simulink model "receiver_overall_reset"  (Simulink 7.5)
settings: Solver=FixedStepDiscrete  SolverMode=SingleTasking  StartTime=0.0  StopTime=(length(simin.signals.values)-1)/Fs  FixedStep=1  RelTol=1e-3
undefined symbols (not defined in the file): Fs
libraries: xbsIndex_r4 x962
(part 6 of 9)

== system receiver_overall_reset/Receiver/Sym-Clk/Corr/Delay_Line/DE16 ==
  In1 : Inport
  1to2 : Subsystem
  DE : xbsIndex_r4/Delay  en=off  latency=1  dbl_ovrd=off  reg_retiming=off  block_type=delay
      settings: xl_area=[1 1 0 0 0 0 0]  block_version=12.1
  Out1 : Outport
  Out2 : Outport  Port=2
  wires:
  1to2/2(Out2) -> Out2/1
  1to2/1(Out1) -> Out1/1
  In1/1 -> DE/1
  DE/1 -> 1to2/1(In)

== system receiver_overall_reset/Receiver/Sym-Clk/Corr/Delay_Line/DE17 ==
  In1 : Inport
  1to2 : Subsystem
  DE : xbsIndex_r4/Delay  en=off  latency=1  dbl_ovrd=off  reg_retiming=off  block_type=delay
      settings: xl_area=[1 1 0 0 0 0 0]  block_version=12.1
  Out1 : Outport
  Out2 : Outport  Port=2
  wires:
  1to2/2(Out2) -> Out2/1
  1to2/1(Out1) -> Out1/1
  In1/1 -> DE/1
  DE/1 -> 1to2/1(In)

== system receiver_overall_reset/Receiver/Sym-Clk/Corr/Delay_Line/DE18 ==
  In1 : Inport
  1to2 : Subsystem
  DE : xbsIndex_r4/Delay  en=off  latency=1  dbl_ovrd=off  reg_retiming=off  block_type=delay
      settings: xl_area=[1 1 0 0 0 0 0]  block_version=12.1
  Out1 : Outport
  Out2 : Outport  Port=2
  wires:
  1to2/2(Out2) -> Out2/1
  1to2/1(Out1) -> Out1/1
  In1/1 -> DE/1
  DE/1 -> 1to2/1(In)

== system receiver_overall_reset/Receiver/Sym-Clk/Corr/Delay_Line/DE19 ==
  In1 : Inport
  1to2 : Subsystem
  DE : xbsIndex_r4/Delay  en=off  latency=1  dbl_ovrd=off  reg_retiming=off  block_type=delay
      settings: xl_area=[1 1 0 0 0 0 0]  block_version=12.1
  Out1 : Outport
  Out2 : Outport  Port=2
  wires:
  1to2/2(Out2) -> Out2/1
  1to2/1(Out1) -> Out1/1
  In1/1 -> DE/1
  DE/1 -> 1to2/1(In)

== system receiver_overall_reset/Receiver/Sym-Clk/Corr/Delay_Line/DE2 ==
  In1 : Inport
  1to2 : Subsystem
  DE : xbsIndex_r4/Delay  en=off  latency=1  dbl_ovrd=off  reg_retiming=off  block_type=delay
      settings: xl_area=[1 1 0 0 0 0 0]  block_version=12.1
  Out1 : Outport
  Out2 : Outport  Port=2
  wires:
  1to2/2(Out2) -> Out2/1
  1to2/1(Out1) -> Out1/1
  In1/1 -> DE/1
  DE/1 -> 1to2/1(In)

== system receiver_overall_reset/Receiver/Sym-Clk/Corr/Delay_Line/DE20 ==
  In1 : Inport
  1to2 : Subsystem
  DE : xbsIndex_r4/Delay  en=off  latency=1  dbl_ovrd=off  reg_retiming=off  block_type=delay
      settings: xl_area=[1 1 0 0 0 0 0]  block_version=12.1
  Out1 : Outport
  Out2 : Outport  Port=2
  wires:
  1to2/2(Out2) -> Out2/1
  1to2/1(Out1) -> Out1/1
  In1/1 -> DE/1
  DE/1 -> 1to2/1(In)

== system receiver_overall_reset/Receiver/Sym-Clk/Corr/Delay_Line/DE21 ==
  In1 : Inport
  1to2 : Subsystem
  DE : xbsIndex_r4/Delay  en=off  latency=1  dbl_ovrd=off  reg_retiming=off  block_type=delay
      settings: xl_area=[1 1 0 0 0 0 0]  block_version=12.1
  Out1 : Outport
  Out2 : Outport  Port=2
  wires:
  1to2/2(Out2) -> Out2/1
  1to2/1(Out1) -> Out1/1
  In1/1 -> DE/1
  DE/1 -> 1to2/1(In)

== system receiver_overall_reset/Receiver/Sym-Clk/Corr/Delay_Line/DE22 ==
  In1 : Inport
  1to2 : Subsystem
  DE : xbsIndex_r4/Delay  en=off  latency=1  dbl_ovrd=off  reg_retiming=off  block_type=delay
      settings: xl_area=[1 1 0 0 0 0 0]  block_version=12.1
  Out1 : Outport
  Out2 : Outport  Port=2
  wires:
  1to2/2(Out2) -> Out2/1
  1to2/1(Out1) -> Out1/1
  In1/1 -> DE/1
  DE/1 -> 1to2/1(In)

== system receiver_overall_reset/Receiver/Sym-Clk/Corr/Delay_Line/DE23 ==
  In1 : Inport
  1to2 : Subsystem
  DE : xbsIndex_r4/Delay  en=off  latency=1  dbl_ovrd=off  reg_retiming=off  block_type=delay
      settings: xl_area=[1 1 0 0 0 0 0]  block_version=12.1
  Out1 : Outport
  Out2 : Outport  Port=2
  wires:
  1to2/2(Out2) -> Out2/1
  1to2/1(Out1) -> Out1/1
  In1/1 -> DE/1
  DE/1 -> 1to2/1(In)

== system receiver_overall_reset/Receiver/Sym-Clk/Corr/Delay_Line/DE24 ==
  In1 : Inport
  1to2 : Subsystem
  DE : xbsIndex_r4/Delay  en=off  latency=1  dbl_ovrd=off  reg_retiming=off  block_type=delay
      settings: xl_area=[1 1 0 0 0 0 0]  block_version=12.1
  Out1 : Outport
  Out2 : Outport  Port=2
  wires:
  1to2/2(Out2) -> Out2/1
  1to2/1(Out1) -> Out1/1
  In1/1 -> DE/1
  DE/1 -> 1to2/1(In)

== system receiver_overall_reset/Receiver/Sym-Clk/Corr/Delay_Line/DE25 ==
  In1 : Inport
  1to2 : Subsystem
  DE : xbsIndex_r4/Delay  en=off  latency=1  dbl_ovrd=off  reg_retiming=off  block_type=delay
      settings: xl_area=[1 1 0 0 0 0 0]  block_version=12.1
  Out1 : Outport
  Out2 : Outport  Port=2
  wires:
  1to2/2(Out2) -> Out2/1
  1to2/1(Out1) -> Out1/1
  In1/1 -> DE/1
  DE/1 -> 1to2/1(In)

== system receiver_overall_reset/Receiver/Sym-Clk/Corr/Delay_Line/DE26 ==
  In1 : Inport
  1to2 : Subsystem
  DE : xbsIndex_r4/Delay  en=off  latency=1  dbl_ovrd=off  reg_retiming=off  block_type=delay
      settings: xl_area=[1 1 0 0 0 0 0]  block_version=12.1
  Out1 : Outport
  Out2 : Outport  Port=2
  wires:
  1to2/2(Out2) -> Out2/1
  1to2/1(Out1) -> Out1/1
  In1/1 -> DE/1
  DE/1 -> 1to2/1(In)

== system receiver_overall_reset/Receiver/Sym-Clk/Corr/Delay_Line/DE27 ==
  In1 : Inport
  1to2 : Subsystem
  DE : xbsIndex_r4/Delay  en=off  latency=1  dbl_ovrd=off  reg_retiming=off  block_type=delay
      settings: xl_area=[1 1 0 0 0 0 0]  block_version=12.1
  Out1 : Outport
  Out2 : Outport  Port=2
  wires:
  1to2/2(Out2) -> Out2/1
  1to2/1(Out1) -> Out1/1
  In1/1 -> DE/1
  DE/1 -> 1to2/1(In)

== system receiver_overall_reset/Receiver/Sym-Clk/Corr/Delay_Line/DE28 ==
  In1 : Inport
  1to2 : Subsystem
  DE : xbsIndex_r4/Delay  en=off  latency=1  dbl_ovrd=off  reg_retiming=off  block_type=delay
      settings: xl_area=[1 1 0 0 0 0 0]  block_version=12.1
  Out1 : Outport
  Out2 : Outport  Port=2
  wires:
  1to2/2(Out2) -> Out2/1
  1to2/1(Out1) -> Out1/1
  In1/1 -> DE/1
  DE/1 -> 1to2/1(In)

== system receiver_overall_reset/Receiver/Sym-Clk/Corr/Delay_Line/DE29 ==
  In1 : Inport
  1to2 : Subsystem
  DE : xbsIndex_r4/Delay  en=off  latency=1  dbl_ovrd=off  reg_retiming=off  block_type=delay
      settings: xl_area=[1 1 0 0 0 0 0]  block_version=12.1
  Out1 : Outport
  Out2 : Outport  Port=2
  wires:
  1to2/2(Out2) -> Out2/1
  1to2/1(Out1) -> Out1/1
  In1/1 -> DE/1
  DE/1 -> 1to2/1(In)

== system receiver_overall_reset/Receiver/Sym-Clk/Corr/Delay_Line/DE3 ==
  In1 : Inport
  1to2 : Subsystem
  DE : xbsIndex_r4/Delay  en=off  latency=1  dbl_ovrd=off  reg_retiming=off  block_type=delay
      settings: xl_area=[1 1 0 0 0 0 0]  block_version=12.1
  Out1 : Outport
  Out2 : Outport  Port=2
  wires:
  1to2/2(Out2) -> Out2/1
  1to2/1(Out1) -> Out1/1
  In1/1 -> DE/1
  DE/1 -> 1to2/1(In)

== system receiver_overall_reset/Receiver/Sym-Clk/Corr/Delay_Line/DE30 ==
  In1 : Inport
  1to2 : Subsystem
  DE : xbsIndex_r4/Delay  en=off  latency=1  dbl_ovrd=off  reg_retiming=off  block_type=delay
      settings: xl_area=[1 1 0 0 0 0 0]  block_version=12.1
  Out1 : Outport
  Out2 : Outport  Port=2
  wires:
  1to2/2(Out2) -> Out2/1
  1to2/1(Out1) -> Out1/1
  In1/1 -> DE/1
  DE/1 -> 1to2/1(In)

== system receiver_overall_reset/Receiver/Sym-Clk/Corr/Delay_Line/DE4 ==
  In1 : Inport
  1to2 : Subsystem
  DE : xbsIndex_r4/Delay  en=off  latency=1  dbl_ovrd=off  reg_retiming=off  block_type=delay
      settings: xl_area=[1 1 0 0 0 0 0]  block_version=12.1
  Out1 : Outport
  Out2 : Outport  Port=2
  wires:
  1to2/2(Out2) -> Out2/1
  1to2/1(Out1) -> Out1/1
  In1/1 -> DE/1
  DE/1 -> 1to2/1(In)

== system receiver_overall_reset/Receiver/Sym-Clk/Corr/Delay_Line/DE5 ==
  In1 : Inport
  1to2 : Subsystem
  DE : xbsIndex_r4/Delay  en=off  latency=1  dbl_ovrd=off  reg_retiming=off  block_type=delay
      settings: xl_area=[1 1 0 0 0 0 0]  block_version=12.1
  Out1 : Outport
  Out2 : Outport  Port=2
  wires:
  1to2/2(Out2) -> Out2/1
  1to2/1(Out1) -> Out1/1
  In1/1 -> DE/1
  DE/1 -> 1to2/1(In)

== system receiver_overall_reset/Receiver/Sym-Clk/Corr/Delay_Line/DE6 ==
  In1 : Inport
  1to2 : Subsystem
  DE : xbsIndex_r4/Delay  en=off  latency=1  dbl_ovrd=off  reg_retiming=off  block_type=delay
      settings: xl_area=[1 1 0 0 0 0 0]  block_version=12.1
  Out1 : Outport
  Out2 : Outport  Port=2
  wires:
  1to2/2(Out2) -> Out2/1
  1to2/1(Out1) -> Out1/1
  In1/1 -> DE/1
  DE/1 -> 1to2/1(In)

== system receiver_overall_reset/Receiver/Sym-Clk/Corr/Delay_Line/DE7 ==
  In1 : Inport
  1to2 : Subsystem
  DE : xbsIndex_r4/Delay  en=off  latency=1  dbl_ovrd=off  reg_retiming=off  block_type=delay
      settings: xl_area=[1 1 0 0 0 0 0]  block_version=12.1
  Out1 : Outport
  Out2 : Outport  Port=2
  wires:
  1to2/2(Out2) -> Out2/1
  1to2/1(Out1) -> Out1/1
  In1/1 -> DE/1
  DE/1 -> 1to2/1(In)

== system receiver_overall_reset/Receiver/Sym-Clk/Corr/Delay_Line/DE8 ==
  In1 : Inport
  1to2 : Subsystem
  DE : xbsIndex_r4/Delay  en=off  latency=1  dbl_ovrd=off  reg_retiming=off  block_type=delay
      settings: xl_area=[1 1 0 0 0 0 0]  block_version=12.1
  Out1 : Outport
  Out2 : Outport  Port=2
  wires:
  1to2/2(Out2) -> Out2/1
  1to2/1(Out1) -> Out1/1
  In1/1 -> DE/1
  DE/1 -> 1to2/1(In)

== system receiver_overall_reset/Receiver/Sym-Clk/Corr/Delay_Line/DE9 ==
  In1 : Inport
  1to2 : Subsystem
  DE : xbsIndex_r4/Delay  en=off  latency=1  dbl_ovrd=off  reg_retiming=off  block_type=delay
      settings: xl_area=[1 1 0 0 0 0 0]  block_version=12.1
  Out1 : Outport
  Out2 : Outport  Port=2
  wires:
  1to2/2(Out2) -> Out2/1
  1to2/1(Out1) -> Out1/1
  In1/1 -> DE/1
  DE/1 -> 1to2/1(In)

== system receiver_overall_reset/Receiver/Sym-Chooser/0-8/Corr0/Delay_Line/1to2 ==
  In : Inport  OutDataType=fixdt(1, 16)  OutScaling=2^0
  Out1 : Outport  OutDataType=fixdt(1, 16)  OutScaling=2^0
  Out2 : Outport  Port=2  OutDataType=fixdt(1, 16)  OutScaling=2^0
  wires:
  In/1 -> Out1/1, Out2/1

== system receiver_overall_reset/Receiver/Sym-Chooser/0-8/Corr0/Delay_Line/DE1 ==
  In1 : Inport
  1to2 : Subsystem
  DE : xbsIndex_r4/Delay  en=off  latency=1  dbl_ovrd=off  reg_retiming=off  block_type=delay
      settings: xl_area=[1 1 0 0 0 0 0]  block_version=12.1
  Out1 : Outport
  Out2 : Outport  Port=2
  wires:
  DE/1 -> 1to2/1(In)
  In1/1 -> DE/1
  1to2/1(Out1) -> Out1/1
  1to2/2(Out2) -> Out2/1

== system receiver_overall_reset/Receiver/Sym-Chooser/0-8/Corr0/Delay_Line/DE10 ==
  In1 : Inport
  1to2 : Subsystem
  DE : xbsIndex_r4/Delay  en=off  latency=1  dbl_ovrd=off  reg_retiming=off  block_type=delay
      settings: xl_area=[1 1 0 0 0 0 0]  block_version=12.1
  Out1 : Outport
  Out2 : Outport  Port=2
  wires:
  1to2/2(Out2) -> Out2/1
  1to2/1(Out1) -> Out1/1
  In1/1 -> DE/1
  DE/1 -> 1to2/1(In)

== system receiver_overall_reset/Receiver/Sym-Chooser/0-8/Corr0/Delay_Line/DE11 ==
  In1 : Inport
  1to2 : Subsystem
  DE : xbsIndex_r4/Delay  en=off  latency=1  dbl_ovrd=off  reg_retiming=off  block_type=delay
      settings: xl_area=[1 1 0 0 0 0 0]  block_version=12.1
  Out1 : Outport
  Out2 : Outport  Port=2
  wires:
  1to2/2(Out2) -> Out2/1
  1to2/1(Out1) -> Out1/1
  In1/1 -> DE/1
  DE/1 -> 1to2/1(In)

== system receiver_overall_reset/Receiver/Sym-Chooser/0-8/Corr0/Delay_Line/DE12 ==
  In1 : Inport
  1to2 : Subsystem
  DE : xbsIndex_r4/Delay  en=off  latency=1  dbl_ovrd=off  reg_retiming=off  block_type=delay
      settings: xl_area=[1 1 0 0 0 0 0]  block_version=12.1
  Out1 : Outport
  Out2 : Outport  Port=2
  wires:
  1to2/2(Out2) -> Out2/1
  1to2/1(Out1) -> Out1/1
  In1/1 -> DE/1
  DE/1 -> 1to2/1(In)

== system receiver_overall_reset/Receiver/Sym-Chooser/0-8/Corr0/Delay_Line/DE13 ==
  In1 : Inport
  1to2 : Subsystem
  DE : xbsIndex_r4/Delay  en=off  latency=1  dbl_ovrd=off  reg_retiming=off  block_type=delay
      settings: xl_area=[1 1 0 0 0 0 0]  block_version=12.1
  Out1 : Outport
  Out2 : Outport  Port=2
  wires:
  1to2/2(Out2) -> Out2/1
  1to2/1(Out1) -> Out1/1
  In1/1 -> DE/1
  DE/1 -> 1to2/1(In)

== system receiver_overall_reset/Receiver/Sym-Chooser/0-8/Corr0/Delay_Line/DE14 ==
  In1 : Inport
  1to2 : Subsystem
  DE : xbsIndex_r4/Delay  en=off  latency=1  dbl_ovrd=off  reg_retiming=off  block_type=delay
      settings: xl_area=[1 1 0 0 0 0 0]  block_version=12.1
  Out1 : Outport
  Out2 : Outport  Port=2
  wires:
  1to2/2(Out2) -> Out2/1
  1to2/1(Out1) -> Out1/1
  In1/1 -> DE/1
  DE/1 -> 1to2/1(In)

== system receiver_overall_reset/Receiver/Sym-Chooser/0-8/Corr0/Delay_Line/DE15 ==
  In1 : Inport
  1to2 : Subsystem
  DE : xbsIndex_r4/Delay  en=off  latency=1  dbl_ovrd=off  reg_retiming=off  block_type=delay
      settings: xl_area=[1 1 0 0 0 0 0]  block_version=12.1
  Out1 : Outport
  Out2 : Outport  Port=2
  wires:
  1to2/2(Out2) -> Out2/1
  1to2/1(Out1) -> Out1/1
  In1/1 -> DE/1
  DE/1 -> 1to2/1(In)

== system receiver_overall_reset/Receiver/Sym-Chooser/0-8/Corr0/Delay_Line/DE16 ==
  In1 : Inport
  1to2 : Subsystem
  DE : xbsIndex_r4/Delay  en=off  latency=1  dbl_ovrd=off  reg_retiming=off  block_type=delay
      settings: xl_area=[1 1 0 0 0 0 0]  block_version=12.1
  Out1 : Outport
  Out2 : Outport  Port=2
  wires:
  1to2/2(Out2) -> Out2/1
  1to2/1(Out1) -> Out1/1
  In1/1 -> DE/1
  DE/1 -> 1to2/1(In)

== system receiver_overall_reset/Receiver/Sym-Chooser/0-8/Corr0/Delay_Line/DE17 ==
  In1 : Inport
  1to2 : Subsystem
  DE : xbsIndex_r4/Delay  en=off  latency=1  dbl_ovrd=off  reg_retiming=off  block_type=delay
      settings: xl_area=[1 1 0 0 0 0 0]  block_version=12.1
  Out1 : Outport
  Out2 : Outport  Port=2
  wires:
  1to2/2(Out2) -> Out2/1
  1to2/1(Out1) -> Out1/1
  In1/1 -> DE/1
  DE/1 -> 1to2/1(In)

== system receiver_overall_reset/Receiver/Sym-Chooser/0-8/Corr0/Delay_Line/DE18 ==
  In1 : Inport
  1to2 : Subsystem
  DE : xbsIndex_r4/Delay  en=off  latency=1  dbl_ovrd=off  reg_retiming=off  block_type=delay
      settings: xl_area=[1 1 0 0 0 0 0]  block_version=12.1
  Out1 : Outport
  Out2 : Outport  Port=2
  wires:
  1to2/2(Out2) -> Out2/1
  1to2/1(Out1) -> Out1/1
  In1/1 -> DE/1
  DE/1 -> 1to2/1(In)

== system receiver_overall_reset/Receiver/Sym-Chooser/0-8/Corr0/Delay_Line/DE19 ==
  In1 : Inport
  1to2 : Subsystem
  DE : xbsIndex_r4/Delay  en=off  latency=1  dbl_ovrd=off  reg_retiming=off  block_type=delay
      settings: xl_area=[1 1 0 0 0 0 0]  block_version=12.1
  Out1 : Outport
  Out2 : Outport  Port=2
  wires:
  1to2/2(Out2) -> Out2/1
  1to2/1(Out1) -> Out1/1
  In1/1 -> DE/1
  DE/1 -> 1to2/1(In)

== system receiver_overall_reset/Receiver/Sym-Chooser/0-8/Corr0/Delay_Line/DE2 ==
  In1 : Inport
  1to2 : Subsystem
  DE : xbsIndex_r4/Delay  en=off  latency=1  dbl_ovrd=off  reg_retiming=off  block_type=delay
      settings: xl_area=[1 1 0 0 0 0 0]  block_version=12.1
  Out1 : Outport
  Out2 : Outport  Port=2
  wires:
  1to2/2(Out2) -> Out2/1
  1to2/1(Out1) -> Out1/1
  In1/1 -> DE/1
  DE/1 -> 1to2/1(In)

== system receiver_overall_reset/Receiver/Sym-Chooser/0-8/Corr0/Delay_Line/DE20 ==
  In1 : Inport
  1to2 : Subsystem
  DE : xbsIndex_r4/Delay  en=off  latency=1  dbl_ovrd=off  reg_retiming=off  block_type=delay
      settings: xl_area=[1 1 0 0 0 0 0]  block_version=12.1
  Out1 : Outport
  Out2 : Outport  Port=2
  wires:
  1to2/2(Out2) -> Out2/1
  1to2/1(Out1) -> Out1/1
  In1/1 -> DE/1
  DE/1 -> 1to2/1(In)

== system receiver_overall_reset/Receiver/Sym-Chooser/0-8/Corr0/Delay_Line/DE21 ==
  In1 : Inport
  1to2 : Subsystem
  DE : xbsIndex_r4/Delay  en=off  latency=1  dbl_ovrd=off  reg_retiming=off  block_type=delay
      settings: xl_area=[1 1 0 0 0 0 0]  block_version=12.1
  Out1 : Outport
  Out2 : Outport  Port=2
  wires:
  1to2/2(Out2) -> Out2/1
  1to2/1(Out1) -> Out1/1
  In1/1 -> DE/1
  DE/1 -> 1to2/1(In)

== system receiver_overall_reset/Receiver/Sym-Chooser/0-8/Corr0/Delay_Line/DE22 ==
  In1 : Inport
  1to2 : Subsystem
  DE : xbsIndex_r4/Delay  en=off  latency=1  dbl_ovrd=off  reg_retiming=off  block_type=delay
      settings: xl_area=[1 1 0 0 0 0 0]  block_version=12.1
  Out1 : Outport
  Out2 : Outport  Port=2
  wires:
  1to2/2(Out2) -> Out2/1
  1to2/1(Out1) -> Out1/1
  In1/1 -> DE/1
  DE/1 -> 1to2/1(In)

== system receiver_overall_reset/Receiver/Sym-Chooser/0-8/Corr0/Delay_Line/DE23 ==
  In1 : Inport
  1to2 : Subsystem
  DE : xbsIndex_r4/Delay  en=off  latency=1  dbl_ovrd=off  reg_retiming=off  block_type=delay
      settings: xl_area=[1 1 0 0 0 0 0]  block_version=12.1
  Out1 : Outport
  Out2 : Outport  Port=2
  wires:
  1to2/2(Out2) -> Out2/1
  1to2/1(Out1) -> Out1/1
  In1/1 -> DE/1
  DE/1 -> 1to2/1(In)

== system receiver_overall_reset/Receiver/Sym-Chooser/0-8/Corr0/Delay_Line/DE24 ==
  In1 : Inport
  1to2 : Subsystem
  DE : xbsIndex_r4/Delay  en=off  latency=1  dbl_ovrd=off  reg_retiming=off  block_type=delay
      settings: xl_area=[1 1 0 0 0 0 0]  block_version=12.1
  Out1 : Outport
  Out2 : Outport  Port=2
  wires:
  1to2/2(Out2) -> Out2/1
  1to2/1(Out1) -> Out1/1
  In1/1 -> DE/1
  DE/1 -> 1to2/1(In)

== system receiver_overall_reset/Receiver/Sym-Chooser/0-8/Corr0/Delay_Line/DE25 ==
  In1 : Inport
  1to2 : Subsystem
  DE : xbsIndex_r4/Delay  en=off  latency=1  dbl_ovrd=off  reg_retiming=off  block_type=delay
      settings: xl_area=[1 1 0 0 0 0 0]  block_version=12.1
  Out1 : Outport
  Out2 : Outport  Port=2
  wires:
  1to2/2(Out2) -> Out2/1
  1to2/1(Out1) -> Out1/1
  In1/1 -> DE/1
  DE/1 -> 1to2/1(In)

== system receiver_overall_reset/Receiver/Sym-Chooser/0-8/Corr0/Delay_Line/DE26 ==
  In1 : Inport
  1to2 : Subsystem
  DE : xbsIndex_r4/Delay  en=off  latency=1  dbl_ovrd=off  reg_retiming=off  block_type=delay
      settings: xl_area=[1 1 0 0 0 0 0]  block_version=12.1
  Out1 : Outport
  Out2 : Outport  Port=2
  wires:
  1to2/2(Out2) -> Out2/1
  1to2/1(Out1) -> Out1/1
  In1/1 -> DE/1
  DE/1 -> 1to2/1(In)

== system receiver_overall_reset/Receiver/Sym-Chooser/0-8/Corr0/Delay_Line/DE27 ==
  In1 : Inport
  1to2 : Subsystem
  DE : xbsIndex_r4/Delay  en=off  latency=1  dbl_ovrd=off  reg_retiming=off  block_type=delay
      settings: xl_area=[1 1 0 0 0 0 0]  block_version=12.1
  Out1 : Outport
  Out2 : Outport  Port=2
  wires:
  1to2/2(Out2) -> Out2/1
  1to2/1(Out1) -> Out1/1
  In1/1 -> DE/1
  DE/1 -> 1to2/1(In)

== system receiver_overall_reset/Receiver/Sym-Chooser/0-8/Corr0/Delay_Line/DE28 ==
  In1 : Inport
  1to2 : Subsystem
  DE : xbsIndex_r4/Delay  en=off  latency=1  dbl_ovrd=off  reg_retiming=off  block_type=delay
      settings: xl_area=[1 1 0 0 0 0 0]  block_version=12.1
  Out1 : Outport
  Out2 : Outport  Port=2
  wires:
  1to2/2(Out2) -> Out2/1
  1to2/1(Out1) -> Out1/1
  In1/1 -> DE/1
  DE/1 -> 1to2/1(In)

== system receiver_overall_reset/Receiver/Sym-Chooser/0-8/Corr0/Delay_Line/DE29 ==
  In1 : Inport
  1to2 : Subsystem
  DE : xbsIndex_r4/Delay  en=off  latency=1  dbl_ovrd=off  reg_retiming=off  block_type=delay
      settings: xl_area=[1 1 0 0 0 0 0]  block_version=12.1
  Out1 : Outport
  Out2 : Outport  Port=2
  wires:
  1to2/2(Out2) -> Out2/1
  1to2/1(Out1) -> Out1/1
  In1/1 -> DE/1
  DE/1 -> 1to2/1(In)

== system receiver_overall_reset/Receiver/Sym-Chooser/0-8/Corr0/Delay_Line/DE3 ==
  In1 : Inport
  1to2 : Subsystem
  DE : xbsIndex_r4/Delay  en=off  latency=1  dbl_ovrd=off  reg_retiming=off  block_type=delay
      settings: xl_area=[1 1 0 0 0 0 0]  block_version=12.1
  Out1 : Outport
  Out2 : Outport  Port=2
  wires:
  1to2/2(Out2) -> Out2/1
  1to2/1(Out1) -> Out1/1
  In1/1 -> DE/1
  DE/1 -> 1to2/1(In)

== system receiver_overall_reset/Receiver/Sym-Chooser/0-8/Corr0/Delay_Line/DE30 ==
  In1 : Inport
  1to2 : Subsystem
  DE : xbsIndex_r4/Delay  en=off  latency=1  dbl_ovrd=off  reg_retiming=off  block_type=delay
      settings: xl_area=[1 1 0 0 0 0 0]  block_version=12.1
  Out1 : Outport
  Out2 : Outport  Port=2
  wires:
  1to2/2(Out2) -> Out2/1
  1to2/1(Out1) -> Out1/1
  In1/1 -> DE/1
  DE/1 -> 1to2/1(In)

== system receiver_overall_reset/Receiver/Sym-Chooser/0-8/Corr0/Delay_Line/DE4 ==
  In1 : Inport
  1to2 : Subsystem
  DE : xbsIndex_r4/Delay  en=off  latency=1  dbl_ovrd=off  reg_retiming=off  block_type=delay
      settings: xl_area=[1 1 0 0 0 0 0]  block_version=12.1
  Out1 : Outport
  Out2 : Outport  Port=2
  wires:
  1to2/2(Out2) -> Out2/1
  1to2/1(Out1) -> Out1/1
  In1/1 -> DE/1
  DE/1 -> 1to2/1(In)

== system receiver_overall_reset/Receiver/Sym-Chooser/0-8/Corr0/Delay_Line/DE5 ==
  In1 : Inport
  1to2 : Subsystem
  DE : xbsIndex_r4/Delay  en=off  latency=1  dbl_ovrd=off  reg_retiming=off  block_type=delay
      settings: xl_area=[1 1 0 0 0 0 0]  block_version=12.1
  Out1 : Outport
  Out2 : Outport  Port=2
  wires:
  1to2/2(Out2) -> Out2/1
  1to2/1(Out1) -> Out1/1
  In1/1 -> DE/1
  DE/1 -> 1to2/1(In)

== system receiver_overall_reset/Receiver/Sym-Chooser/0-8/Corr0/Delay_Line/DE6 ==
  In1 : Inport
  1to2 : Subsystem
  DE : xbsIndex_r4/Delay  en=off  latency=1  dbl_ovrd=off  reg_retiming=off  block_type=delay
      settings: xl_area=[1 1 0 0 0 0 0]  block_version=12.1
  Out1 : Outport
  Out2 : Outport  Port=2
  wires:
  1to2/2(Out2) -> Out2/1
  1to2/1(Out1) -> Out1/1
  In1/1 -> DE/1
  DE/1 -> 1to2/1(In)

== system receiver_overall_reset/Receiver/Sym-Chooser/0-8/Corr0/Delay_Line/DE7 ==
  In1 : Inport
  1to2 : Subsystem
  DE : xbsIndex_r4/Delay  en=off  latency=1  dbl_ovrd=off  reg_retiming=off  block_type=delay
      settings: xl_area=[1 1 0 0 0 0 0]  block_version=12.1
  Out1 : Outport
  Out2 : Outport  Port=2
  wires:
  1to2/2(Out2) -> Out2/1
  1to2/1(Out1) -> Out1/1
  In1/1 -> DE/1
  DE/1 -> 1to2/1(In)

== system receiver_overall_reset/Receiver/Sym-Chooser/0-8/Corr0/Delay_Line/DE8 ==
  In1 : Inport
  1to2 : Subsystem
  DE : xbsIndex_r4/Delay  en=off  latency=1  dbl_ovrd=off  reg_retiming=off  block_type=delay
      settings: xl_area=[1 1 0 0 0 0 0]  block_version=12.1
  Out1 : Outport
  Out2 : Outport  Port=2
  wires:
  1to2/2(Out2) -> Out2/1
  1to2/1(Out1) -> Out1/1
  In1/1 -> DE/1
  DE/1 -> 1to2/1(In)

== system receiver_overall_reset/Receiver/Sym-Chooser/0-8/Corr0/Delay_Line/DE9 ==
  In1 : Inport
  1to2 : Subsystem
  DE : xbsIndex_r4/Delay  en=off  latency=1  dbl_ovrd=off  reg_retiming=off  block_type=delay
      settings: xl_area=[1 1 0 0 0 0 0]  block_version=12.1
  Out1 : Outport
  Out2 : Outport  Port=2
  wires:
  1to2/2(Out2) -> Out2/1
  1to2/1(Out1) -> Out1/1
  In1/1 -> DE/1
  DE/1 -> 1to2/1(In)

== system receiver_overall_reset/Receiver/Sym-Chooser/1-9/Corr0/Delay_Line/1to2 ==
  In : Inport  OutDataType=fixdt(1, 16)  OutScaling=2^0
  Out1 : Outport  OutDataType=fixdt(1, 16)  OutScaling=2^0
  Out2 : Outport  Port=2  OutDataType=fixdt(1, 16)  OutScaling=2^0
  wires:
  In/1 -> Out1/1, Out2/1

== system receiver_overall_reset/Receiver/Sym-Chooser/1-9/Corr0/Delay_Line/DE1 ==
  In1 : Inport
  1to2 : Subsystem
  DE : xbsIndex_r4/Delay  en=off  latency=1  dbl_ovrd=off  reg_retiming=off  block_type=delay
      settings: xl_area=[1 1 0 0 0 0 0]  block_version=12.1
  Out1 : Outport
  Out2 : Outport  Port=2
  wires:
  DE/1 -> 1to2/1(In)
  In1/1 -> DE/1
  1to2/1(Out1) -> Out1/1
  1to2/2(Out2) -> Out2/1

== system receiver_overall_reset/Receiver/Sym-Chooser/1-9/Corr0/Delay_Line/DE10 ==
  In1 : Inport
  1to2 : Subsystem
  DE : xbsIndex_r4/Delay  en=off  latency=1  dbl_ovrd=off  reg_retiming=off  block_type=delay
      settings: xl_area=[1 1 0 0 0 0 0]  block_version=12.1
  Out1 : Outport
  Out2 : Outport  Port=2
  wires:
  1to2/2(Out2) -> Out2/1
  1to2/1(Out1) -> Out1/1
  In1/1 -> DE/1
  DE/1 -> 1to2/1(In)

== system receiver_overall_reset/Receiver/Sym-Chooser/1-9/Corr0/Delay_Line/DE11 ==
  In1 : Inport
  1to2 : Subsystem
  DE : xbsIndex_r4/Delay  en=off  latency=1  dbl_ovrd=off  reg_retiming=off  block_type=delay
      settings: xl_area=[1 1 0 0 0 0 0]  block_version=12.1
  Out1 : Outport
  Out2 : Outport  Port=2
  wires:
  1to2/2(Out2) -> Out2/1
  1to2/1(Out1) -> Out1/1
  In1/1 -> DE/1
  DE/1 -> 1to2/1(In)

== system receiver_overall_reset/Receiver/Sym-Chooser/1-9/Corr0/Delay_Line/DE12 ==
  In1 : Inport
  1to2 : Subsystem
  DE : xbsIndex_r4/Delay  en=off  latency=1  dbl_ovrd=off  reg_retiming=off  block_type=delay
      settings: xl_area=[1 1 0 0 0 0 0]  block_version=12.1
  Out1 : Outport
  Out2 : Outport  Port=2
  wires:
  1to2/2(Out2) -> Out2/1
  1to2/1(Out1) -> Out1/1
  In1/1 -> DE/1
  DE/1 -> 1to2/1(In)

== system receiver_overall_reset/Receiver/Sym-Chooser/1-9/Corr0/Delay_Line/DE13 ==
  In1 : Inport
  1to2 : Subsystem
  DE : xbsIndex_r4/Delay  en=off  latency=1  dbl_ovrd=off  reg_retiming=off  block_type=delay
      settings: xl_area=[1 1 0 0 0 0 0]  block_version=12.1
  Out1 : Outport
  Out2 : Outport  Port=2
  wires:
  1to2/2(Out2) -> Out2/1
  1to2/1(Out1) -> Out1/1
  In1/1 -> DE/1
  DE/1 -> 1to2/1(In)

== system receiver_overall_reset/Receiver/Sym-Chooser/1-9/Corr0/Delay_Line/DE14 ==
  In1 : Inport
  1to2 : Subsystem
  DE : xbsIndex_r4/Delay  en=off  latency=1  dbl_ovrd=off  reg_retiming=off  block_type=delay
      settings: xl_area=[1 1 0 0 0 0 0]  block_version=12.1
  Out1 : Outport
  Out2 : Outport  Port=2
  wires:
  1to2/2(Out2) -> Out2/1
  1to2/1(Out1) -> Out1/1
  In1/1 -> DE/1
  DE/1 -> 1to2/1(In)

== system receiver_overall_reset/Receiver/Sym-Chooser/1-9/Corr0/Delay_Line/DE15 ==
  In1 : Inport
  1to2 : Subsystem
  DE : xbsIndex_r4/Delay  en=off  latency=1  dbl_ovrd=off  reg_retiming=off  block_type=delay
      settings: xl_area=[1 1 0 0 0 0 0]  block_version=12.1
  Out1 : Outport
  Out2 : Outport  Port=2
  wires:
  1to2/2(Out2) -> Out2/1
  1to2/1(Out1) -> Out1/1
  In1/1 -> DE/1
  DE/1 -> 1to2/1(In)

== system receiver_overall_reset/Receiver/Sym-Chooser/1-9/Corr0/Delay_Line/DE16 ==
  In1 : Inport
  1to2 : Subsystem
  DE : xbsIndex_r4/Delay  en=off  latency=1  dbl_ovrd=off  reg_retiming=off  block_type=delay
      settings: xl_area=[1 1 0 0 0 0 0]  block_version=12.1
  Out1 : Outport
  Out2 : Outport  Port=2
  wires:
  1to2/2(Out2) -> Out2/1
  1to2/1(Out1) -> Out1/1
  In1/1 -> DE/1
  DE/1 -> 1to2/1(In)

== system receiver_overall_reset/Receiver/Sym-Chooser/1-9/Corr0/Delay_Line/DE17 ==
  In1 : Inport
  1to2 : Subsystem
  DE : xbsIndex_r4/Delay  en=off  latency=1  dbl_ovrd=off  reg_retiming=off  block_type=delay
      settings: xl_area=[1 1 0 0 0 0 0]  block_version=12.1
  Out1 : Outport
  Out2 : Outport  Port=2
  wires:
  1to2/2(Out2) -> Out2/1
  1to2/1(Out1) -> Out1/1
  In1/1 -> DE/1
  DE/1 -> 1to2/1(In)

== system receiver_overall_reset/Receiver/Sym-Chooser/1-9/Corr0/Delay_Line/DE18 ==
  In1 : Inport
  1to2 : Subsystem
  DE : xbsIndex_r4/Delay  en=off  latency=1  dbl_ovrd=off  reg_retiming=off  block_type=delay
      settings: xl_area=[1 1 0 0 0 0 0]  block_version=12.1
  Out1 : Outport
  Out2 : Outport  Port=2
  wires:
  1to2/2(Out2) -> Out2/1
  1to2/1(Out1) -> Out1/1
  In1/1 -> DE/1
  DE/1 -> 1to2/1(In)

== system receiver_overall_reset/Receiver/Sym-Chooser/1-9/Corr0/Delay_Line/DE19 ==
  In1 : Inport
  1to2 : Subsystem
  DE : xbsIndex_r4/Delay  en=off  latency=1  dbl_ovrd=off  reg_retiming=off  block_type=delay
      settings: xl_area=[1 1 0 0 0 0 0]  block_version=12.1
  Out1 : Outport
  Out2 : Outport  Port=2
  wires:
  1to2/2(Out2) -> Out2/1
  1to2/1(Out1) -> Out1/1
  In1/1 -> DE/1
  DE/1 -> 1to2/1(In)

== system receiver_overall_reset/Receiver/Sym-Chooser/1-9/Corr0/Delay_Line/DE2 ==
  In1 : Inport
  1to2 : Subsystem
  DE : xbsIndex_r4/Delay  en=off  latency=1  dbl_ovrd=off  reg_retiming=off  block_type=delay
      settings: xl_area=[1 1 0 0 0 0 0]  block_version=12.1
  Out1 : Outport
  Out2 : Outport  Port=2
  wires:
  1to2/2(Out2) -> Out2/1
  1to2/1(Out1) -> Out1/1
  In1/1 -> DE/1
  DE/1 -> 1to2/1(In)

== system receiver_overall_reset/Receiver/Sym-Chooser/1-9/Corr0/Delay_Line/DE20 ==
  In1 : Inport
  1to2 : Subsystem
  DE : xbsIndex_r4/Delay  en=off  latency=1  dbl_ovrd=off  reg_retiming=off  block_type=delay
      settings: xl_area=[1 1 0 0 0 0 0]  block_version=12.1
  Out1 : Outport
  Out2 : Outport  Port=2
  wires:
  1to2/2(Out2) -> Out2/1
  1to2/1(Out1) -> Out1/1
  In1/1 -> DE/1
  DE/1 -> 1to2/1(In)

== system receiver_overall_reset/Receiver/Sym-Chooser/1-9/Corr0/Delay_Line/DE21 ==
  In1 : Inport
  1to2 : Subsystem
  DE : xbsIndex_r4/Delay  en=off  latency=1  dbl_ovrd=off  reg_retiming=off  block_type=delay
      settings: xl_area=[1 1 0 0 0 0 0]  block_version=12.1
  Out1 : Outport
  Out2 : Outport  Port=2
  wires:
  1to2/2(Out2) -> Out2/1
  1to2/1(Out1) -> Out1/1
  In1/1 -> DE/1
  DE/1 -> 1to2/1(In)

== system receiver_overall_reset/Receiver/Sym-Chooser/1-9/Corr0/Delay_Line/DE22 ==
  In1 : Inport
  1to2 : Subsystem
  DE : xbsIndex_r4/Delay  en=off  latency=1  dbl_ovrd=off  reg_retiming=off  block_type=delay
      settings: xl_area=[1 1 0 0 0 0 0]  block_version=12.1
  Out1 : Outport
  Out2 : Outport  Port=2
  wires:
  1to2/2(Out2) -> Out2/1
  1to2/1(Out1) -> Out1/1
  In1/1 -> DE/1
  DE/1 -> 1to2/1(In)

== system receiver_overall_reset/Receiver/Sym-Chooser/1-9/Corr0/Delay_Line/DE23 ==
  In1 : Inport
  1to2 : Subsystem
  DE : xbsIndex_r4/Delay  en=off  latency=1  dbl_ovrd=off  reg_retiming=off  block_type=delay
      settings: xl_area=[1 1 0 0 0 0 0]  block_version=12.1
  Out1 : Outport
  Out2 : Outport  Port=2
  wires:
  1to2/2(Out2) -> Out2/1
  1to2/1(Out1) -> Out1/1
  In1/1 -> DE/1
  DE/1 -> 1to2/1(In)

== system receiver_overall_reset/Receiver/Sym-Chooser/1-9/Corr0/Delay_Line/DE24 ==
  In1 : Inport
  1to2 : Subsystem
  DE : xbsIndex_r4/Delay  en=off  latency=1  dbl_ovrd=off  reg_retiming=off  block_type=delay
      settings: xl_area=[1 1 0 0 0 0 0]  block_version=12.1
  Out1 : Outport
  Out2 : Outport  Port=2
  wires:
  1to2/2(Out2) -> Out2/1
  1to2/1(Out1) -> Out1/1
  In1/1 -> DE/1
  DE/1 -> 1to2/1(In)

== system receiver_overall_reset/Receiver/Sym-Chooser/1-9/Corr0/Delay_Line/DE25 ==
  In1 : Inport
  1to2 : Subsystem
  DE : xbsIndex_r4/Delay  en=off  latency=1  dbl_ovrd=off  reg_retiming=off  block_type=delay
      settings: xl_area=[1 1 0 0 0 0 0]  block_version=12.1
  Out1 : Outport
  Out2 : Outport  Port=2
  wires:
  1to2/2(Out2) -> Out2/1
  1to2/1(Out1) -> Out1/1
  In1/1 -> DE/1
  DE/1 -> 1to2/1(In)

== system receiver_overall_reset/Receiver/Sym-Chooser/1-9/Corr0/Delay_Line/DE26 ==
  In1 : Inport
  1to2 : Subsystem
  DE : xbsIndex_r4/Delay  en=off  latency=1  dbl_ovrd=off  reg_retiming=off  block_type=delay
      settings: xl_area=[1 1 0 0 0 0 0]  block_version=12.1
  Out1 : Outport
  Out2 : Outport  Port=2
  wires:
  1to2/2(Out2) -> Out2/1
  1to2/1(Out1) -> Out1/1
  In1/1 -> DE/1
  DE/1 -> 1to2/1(In)

== system receiver_overall_reset/Receiver/Sym-Chooser/1-9/Corr0/Delay_Line/DE27 ==
  In1 : Inport
  1to2 : Subsystem
  DE : xbsIndex_r4/Delay  en=off  latency=1  dbl_ovrd=off  reg_retiming=off  block_type=delay
      settings: xl_area=[1 1 0 0 0 0 0]  block_version=12.1
  Out1 : Outport
  Out2 : Outport  Port=2
  wires:
  1to2/2(Out2) -> Out2/1
  1to2/1(Out1) -> Out1/1
  In1/1 -> DE/1
  DE/1 -> 1to2/1(In)

== system receiver_overall_reset/Receiver/Sym-Chooser/1-9/Corr0/Delay_Line/DE28 ==
  In1 : Inport
  1to2 : Subsystem
  DE : xbsIndex_r4/Delay  en=off  latency=1  dbl_ovrd=off  reg_retiming=off  block_type=delay
      settings: xl_area=[1 1 0 0 0 0 0]  block_version=12.1
  Out1 : Outport
  Out2 : Outport  Port=2
  wires:
  1to2/2(Out2) -> Out2/1
  1to2/1(Out1) -> Out1/1
  In1/1 -> DE/1
  DE/1 -> 1to2/1(In)

== system receiver_overall_reset/Receiver/Sym-Chooser/1-9/Corr0/Delay_Line/DE29 ==
  In1 : Inport
  1to2 : Subsystem
  DE : xbsIndex_r4/Delay  en=off  latency=1  dbl_ovrd=off  reg_retiming=off  block_type=delay
      settings: xl_area=[1 1 0 0 0 0 0]  block_version=12.1
  Out1 : Outport
  Out2 : Outport  Port=2
  wires:
  1to2/2(Out2) -> Out2/1
  1to2/1(Out1) -> Out1/1
  In1/1 -> DE/1
  DE/1 -> 1to2/1(In)

== system receiver_overall_reset/Receiver/Sym-Chooser/1-9/Corr0/Delay_Line/DE3 ==
  In1 : Inport
  1to2 : Subsystem
  DE : xbsIndex_r4/Delay  en=off  latency=1  dbl_ovrd=off  reg_retiming=off  block_type=delay
      settings: xl_area=[1 1 0 0 0 0 0]  block_version=12.1
  Out1 : Outport
  Out2 : Outport  Port=2
  wires:
  1to2/2(Out2) -> Out2/1
  1to2/1(Out1) -> Out1/1
  In1/1 -> DE/1
  DE/1 -> 1to2/1(In)

== system receiver_overall_reset/Receiver/Sym-Chooser/1-9/Corr0/Delay_Line/DE30 ==
  In1 : Inport
  1to2 : Subsystem
  DE : xbsIndex_r4/Delay  en=off  latency=1  dbl_ovrd=off  reg_retiming=off  block_type=delay
      settings: xl_area=[1 1 0 0 0 0 0]  block_version=12.1
  Out1 : Outport
  Out2 : Outport  Port=2
  wires:
  1to2/2(Out2) -> Out2/1
  1to2/1(Out1) -> Out1/1
  In1/1 -> DE/1
  DE/1 -> 1to2/1(In)

== system receiver_overall_reset/Receiver/Sym-Chooser/1-9/Corr0/Delay_Line/DE4 ==
  In1 : Inport
  1to2 : Subsystem
  DE : xbsIndex_r4/Delay  en=off  latency=1  dbl_ovrd=off  reg_retiming=off  block_type=delay
      settings: xl_area=[1 1 0 0 0 0 0]  block_version=12.1
  Out1 : Outport
  Out2 : Outport  Port=2
  wires:
  1to2/2(Out2) -> Out2/1
  1to2/1(Out1) -> Out1/1
  In1/1 -> DE/1
  DE/1 -> 1to2/1(In)

== system receiver_overall_reset/Receiver/Sym-Chooser/1-9/Corr0/Delay_Line/DE5 ==
  In1 : Inport
  1to2 : Subsystem
  DE : xbsIndex_r4/Delay  en=off  latency=1  dbl_ovrd=off  reg_retiming=off  block_type=delay
      settings: xl_area=[1 1 0 0 0 0 0]  block_version=12.1
  Out1 : Outport
  Out2 : Outport  Port=2
  wires:
  1to2/2(Out2) -> Out2/1
  1to2/1(Out1) -> Out1/1
  In1/1 -> DE/1
  DE/1 -> 1to2/1(In)

== system receiver_overall_reset/Receiver/Sym-Chooser/1-9/Corr0/Delay_Line/DE6 ==
  In1 : Inport
  1to2 : Subsystem
  DE : xbsIndex_r4/Delay  en=off  latency=1  dbl_ovrd=off  reg_retiming=off  block_type=delay
      settings: xl_area=[1 1 0 0 0 0 0]  block_version=12.1
  Out1 : Outport
  Out2 : Outport  Port=2
  wires:
  1to2/2(Out2) -> Out2/1
  1to2/1(Out1) -> Out1/1
  In1/1 -> DE/1
  DE/1 -> 1to2/1(In)

== system receiver_overall_reset/Receiver/Sym-Chooser/1-9/Corr0/Delay_Line/DE7 ==
  In1 : Inport
  1to2 : Subsystem
  DE : xbsIndex_r4/Delay  en=off  latency=1  dbl_ovrd=off  reg_retiming=off  block_type=delay
      settings: xl_area=[1 1 0 0 0 0 0]  block_version=12.1
  Out1 : Outport
  Out2 : Outport  Port=2
  wires:
  1to2/2(Out2) -> Out2/1
  1to2/1(Out1) -> Out1/1
  In1/1 -> DE/1
  DE/1 -> 1to2/1(In)

== system receiver_overall_reset/Receiver/Sym-Chooser/1-9/Corr0/Delay_Line/DE8 ==
  In1 : Inport
  1to2 : Subsystem
  DE : xbsIndex_r4/Delay  en=off  latency=1  dbl_ovrd=off  reg_retiming=off  block_type=delay
      settings: xl_area=[1 1 0 0 0 0 0]  block_version=12.1
  Out1 : Outport
  Out2 : Outport  Port=2
  wires:
  1to2/2(Out2) -> Out2/1
  1to2/1(Out1) -> Out1/1
  In1/1 -> DE/1
  DE/1 -> 1to2/1(In)

== system receiver_overall_reset/Receiver/Sym-Chooser/1-9/Corr0/Delay_Line/DE9 ==
  In1 : Inport
  1to2 : Subsystem
  DE : xbsIndex_r4/Delay  en=off  latency=1  dbl_ovrd=off  reg_retiming=off  block_type=delay
      settings: xl_area=[1 1 0 0 0 0 0]  block_version=12.1
  Out1 : Outport
  Out2 : Outport  Port=2
  wires:
  1to2/2(Out2) -> Out2/1
  1to2/1(Out1) -> Out1/1
  In1/1 -> DE/1
  DE/1 -> 1to2/1(In)

== system receiver_overall_reset/Receiver/Sym-Chooser/2-10/Corr0/Delay_Line/1to2 ==
  In : Inport  OutDataType=fixdt(1, 16)  OutScaling=2^0
  Out1 : Outport  OutDataType=fixdt(1, 16)  OutScaling=2^0
  Out2 : Outport  Port=2  OutDataType=fixdt(1, 16)  OutScaling=2^0
  wires:
  In/1 -> Out1/1, Out2/1

== system receiver_overall_reset/Receiver/Sym-Chooser/2-10/Corr0/Delay_Line/DE1 ==
  In1 : Inport
  1to2 : Subsystem
  DE : xbsIndex_r4/Delay  en=off  latency=1  dbl_ovrd=off  reg_retiming=off  block_type=delay
      settings: xl_area=[1 1 0 0 0 0 0]  block_version=12.1
  Out1 : Outport
  Out2 : Outport  Port=2
  wires:
  DE/1 -> 1to2/1(In)
  In1/1 -> DE/1
  1to2/1(Out1) -> Out1/1
  1to2/2(Out2) -> Out2/1

== system receiver_overall_reset/Receiver/Sym-Chooser/2-10/Corr0/Delay_Line/DE10 ==
  In1 : Inport
  1to2 : Subsystem
  DE : xbsIndex_r4/Delay  en=off  latency=1  dbl_ovrd=off  reg_retiming=off  block_type=delay
      settings: xl_area=[1 1 0 0 0 0 0]  block_version=12.1
  Out1 : Outport
  Out2 : Outport  Port=2
  wires:
  1to2/2(Out2) -> Out2/1
  1to2/1(Out1) -> Out1/1
  In1/1 -> DE/1
  DE/1 -> 1to2/1(In)

== system receiver_overall_reset/Receiver/Sym-Chooser/2-10/Corr0/Delay_Line/DE11 ==
  In1 : Inport
  1to2 : Subsystem
  DE : xbsIndex_r4/Delay  en=off  latency=1  dbl_ovrd=off  reg_retiming=off  block_type=delay
      settings: xl_area=[1 1 0 0 0 0 0]  block_version=12.1
  Out1 : Outport
  Out2 : Outport  Port=2
  wires:
  1to2/2(Out2) -> Out2/1
  1to2/1(Out1) -> Out1/1
  In1/1 -> DE/1
  DE/1 -> 1to2/1(In)

== system receiver_overall_reset/Receiver/Sym-Chooser/2-10/Corr0/Delay_Line/DE12 ==
  In1 : Inport
  1to2 : Subsystem
  DE : xbsIndex_r4/Delay  en=off  latency=1  dbl_ovrd=off  reg_retiming=off  block_type=delay
      settings: xl_area=[1 1 0 0 0 0 0]  block_version=12.1
  Out1 : Outport
  Out2 : Outport  Port=2
  wires:
  1to2/2(Out2) -> Out2/1
  1to2/1(Out1) -> Out1/1
  In1/1 -> DE/1
  DE/1 -> 1to2/1(In)

== system receiver_overall_reset/Receiver/Sym-Chooser/2-10/Corr0/Delay_Line/DE13 ==
  In1 : Inport
  1to2 : Subsystem
  DE : xbsIndex_r4/Delay  en=off  latency=1  dbl_ovrd=off  reg_retiming=off  block_type=delay
      settings: xl_area=[1 1 0 0 0 0 0]  block_version=12.1
  Out1 : Outport
  Out2 : Outport  Port=2
  wires:
  1to2/2(Out2) -> Out2/1
  1to2/1(Out1) -> Out1/1
  In1/1 -> DE/1
  DE/1 -> 1to2/1(In)

== system receiver_overall_reset/Receiver/Sym-Chooser/2-10/Corr0/Delay_Line/DE14 ==
  In1 : Inport
  1to2 : Subsystem
  DE : xbsIndex_r4/Delay  en=off  latency=1  dbl_ovrd=off  reg_retiming=off  block_type=delay
      settings: xl_area=[1 1 0 0 0 0 0]  block_version=12.1
  Out1 : Outport
  Out2 : Outport  Port=2
  wires:
  1to2/2(Out2) -> Out2/1
  1to2/1(Out1) -> Out1/1
  In1/1 -> DE/1
  DE/1 -> 1to2/1(In)

== system receiver_overall_reset/Receiver/Sym-Chooser/2-10/Corr0/Delay_Line/DE15 ==
  In1 : Inport
  1to2 : Subsystem
  DE : xbsIndex_r4/Delay  en=off  latency=1  dbl_ovrd=off  reg_retiming=off  block_type=delay
      settings: xl_area=[1 1 0 0 0 0 0]  block_version=12.1
  Out1 : Outport
  Out2 : Outport  Port=2
  wires:
  1to2/2(Out2) -> Out2/1
  1to2/1(Out1) -> Out1/1
  In1/1 -> DE/1
  DE/1 -> 1to2/1(In)

== system receiver_overall_reset/Receiver/Sym-Chooser/2-10/Corr0/Delay_Line/DE16 ==
  In1 : Inport
  1to2 : Subsystem
  DE : xbsIndex_r4/Delay  en=off  latency=1  dbl_ovrd=off  reg_retiming=off  block_type=delay
      settings: xl_area=[1 1 0 0 0 0 0]  block_version=12.1
  Out1 : Outport
  Out2 : Outport  Port=2
  wires:
  1to2/2(Out2) -> Out2/1
  1to2/1(Out1) -> Out1/1
  In1/1 -> DE/1
  DE/1 -> 1to2/1(In)

== system receiver_overall_reset/Receiver/Sym-Chooser/2-10/Corr0/Delay_Line/DE17 ==
  In1 : Inport
  1to2 : Subsystem
  DE : xbsIndex_r4/Delay  en=off  latency=1  dbl_ovrd=off  reg_retiming=off  block_type=delay
      settings: xl_area=[1 1 0 0 0 0 0]  block_version=12.1
  Out1 : Outport
  Out2 : Outport  Port=2
  wires:
  1to2/2(Out2) -> Out2/1
  1to2/1(Out1) -> Out1/1
  In1/1 -> DE/1
  DE/1 -> 1to2/1(In)

== system receiver_overall_reset/Receiver/Sym-Chooser/2-10/Corr0/Delay_Line/DE18 ==
  In1 : Inport
  1to2 : Subsystem
  DE : xbsIndex_r4/Delay  en=off  latency=1  dbl_ovrd=off  reg_retiming=off  block_type=delay
      settings: xl_area=[1 1 0 0 0 0 0]  block_version=12.1
  Out1 : Outport
  Out2 : Outport  Port=2
  wires:
  1to2/2(Out2) -> Out2/1
  1to2/1(Out1) -> Out1/1
  In1/1 -> DE/1
  DE/1 -> 1to2/1(In)

== system receiver_overall_reset/Receiver/Sym-Chooser/2-10/Corr0/Delay_Line/DE19 ==
  In1 : Inport
  1to2 : Subsystem
  DE : xbsIndex_r4/Delay  en=off  latency=1  dbl_ovrd=off  reg_retiming=off  block_type=delay
      settings: xl_area=[1 1 0 0 0 0 0]  block_version=12.1
  Out1 : Outport
  Out2 : Outport  Port=2
  wires:
  1to2/2(Out2) -> Out2/1
  1to2/1(Out1) -> Out1/1
  In1/1 -> DE/1
  DE/1 -> 1to2/1(In)

== system receiver_overall_reset/Receiver/Sym-Chooser/2-10/Corr0/Delay_Line/DE2 ==
  In1 : Inport
  1to2 : Subsystem
  DE : xbsIndex_r4/Delay  en=off  latency=1  dbl_ovrd=off  reg_retiming=off  block_type=delay
      settings: xl_area=[1 1 0 0 0 0 0]  block_version=12.1
  Out1 : Outport
  Out2 : Outport  Port=2
  wires:
  1to2/2(Out2) -> Out2/1
  1to2/1(Out1) -> Out1/1
  In1/1 -> DE/1
  DE/1 -> 1to2/1(In)

== system receiver_overall_reset/Receiver/Sym-Chooser/2-10/Corr0/Delay_Line/DE20 ==
  In1 : Inport
  1to2 : Subsystem
  DE : xbsIndex_r4/Delay  en=off  latency=1  dbl_ovrd=off  reg_retiming=off  block_type=delay
      settings: xl_area=[1 1 0 0 0 0 0]  block_version=12.1
  Out1 : Outport
  Out2 : Outport  Port=2
  wires:
  1to2/2(Out2) -> Out2/1
  1to2/1(Out1) -> Out1/1
  In1/1 -> DE/1
  DE/1 -> 1to2/1(In)

== system receiver_overall_reset/Receiver/Sym-Chooser/2-10/Corr0/Delay_Line/DE21 ==
  In1 : Inport
  1to2 : Subsystem
  DE : xbsIndex_r4/Delay  en=off  latency=1  dbl_ovrd=off  reg_retiming=off  block_type=delay
      settings: xl_area=[1 1 0 0 0 0 0]  block_version=12.1
  Out1 : Outport
  Out2 : Outport  Port=2
  wires:
  1to2/2(Out2) -> Out2/1
  1to2/1(Out1) -> Out1/1
  In1/1 -> DE/1
  DE/1 -> 1to2/1(In)

== system receiver_overall_reset/Receiver/Sym-Chooser/2-10/Corr0/Delay_Line/DE22 ==
  In1 : Inport
  1to2 : Subsystem
  DE : xbsIndex_r4/Delay  en=off  latency=1  dbl_ovrd=off  reg_retiming=off  block_type=delay
      settings: xl_area=[1 1 0 0 0 0 0]  block_version=12.1
  Out1 : Outport
  Out2 : Outport  Port=2
  wires:
  1to2/2(Out2) -> Out2/1
  1to2/1(Out1) -> Out1/1
  In1/1 -> DE/1
  DE/1 -> 1to2/1(In)

== system receiver_overall_reset/Receiver/Sym-Chooser/2-10/Corr0/Delay_Line/DE23 ==
  In1 : Inport
  1to2 : Subsystem
  DE : xbsIndex_r4/Delay  en=off  latency=1  dbl_ovrd=off  reg_retiming=off  block_type=delay
      settings: xl_area=[1 1 0 0 0 0 0]  block_version=12.1
  Out1 : Outport
  Out2 : Outport  Port=2
  wires:
  1to2/2(Out2) -> Out2/1
  1to2/1(Out1) -> Out1/1
  In1/1 -> DE/1
  DE/1 -> 1to2/1(In)

== system receiver_overall_reset/Receiver/Sym-Chooser/2-10/Corr0/Delay_Line/DE24 ==
  In1 : Inport
  1to2 : Subsystem
  DE : xbsIndex_r4/Delay  en=off  latency=1  dbl_ovrd=off  reg_retiming=off  block_type=delay
      settings: xl_area=[1 1 0 0 0 0 0]  block_version=12.1
  Out1 : Outport
  Out2 : Outport  Port=2
  wires:
  1to2/2(Out2) -> Out2/1
  1to2/1(Out1) -> Out1/1
  In1/1 -> DE/1
  DE/1 -> 1to2/1(In)

== system receiver_overall_reset/Receiver/Sym-Chooser/2-10/Corr0/Delay_Line/DE25 ==
  In1 : Inport
  1to2 : Subsystem
  DE : xbsIndex_r4/Delay  en=off  latency=1  dbl_ovrd=off  reg_retiming=off  block_type=delay
      settings: xl_area=[1 1 0 0 0 0 0]  block_version=12.1
  Out1 : Outport
  Out2 : Outport  Port=2
  wires:
  1to2/2(Out2) -> Out2/1
  1to2/1(Out1) -> Out1/1
  In1/1 -> DE/1
  DE/1 -> 1to2/1(In)

== system receiver_overall_reset/Receiver/Sym-Chooser/2-10/Corr0/Delay_Line/DE26 ==
  In1 : Inport
  1to2 : Subsystem
  DE : xbsIndex_r4/Delay  en=off  latency=1  dbl_ovrd=off  reg_retiming=off  block_type=delay
      settings: xl_area=[1 1 0 0 0 0 0]  block_version=12.1
  Out1 : Outport
  Out2 : Outport  Port=2
  wires:
  1to2/2(Out2) -> Out2/1
  1to2/1(Out1) -> Out1/1
  In1/1 -> DE/1
  DE/1 -> 1to2/1(In)

== system receiver_overall_reset/Receiver/Sym-Chooser/2-10/Corr0/Delay_Line/DE27 ==
  In1 : Inport
  1to2 : Subsystem
  DE : xbsIndex_r4/Delay  en=off  latency=1  dbl_ovrd=off  reg_retiming=off  block_type=delay
      settings: xl_area=[1 1 0 0 0 0 0]  block_version=12.1
  Out1 : Outport
  Out2 : Outport  Port=2
  wires:
  1to2/2(Out2) -> Out2/1
  1to2/1(Out1) -> Out1/1
  In1/1 -> DE/1
  DE/1 -> 1to2/1(In)

== system receiver_overall_reset/Receiver/Sym-Chooser/2-10/Corr0/Delay_Line/DE28 ==
  In1 : Inport
  1to2 : Subsystem
  DE : xbsIndex_r4/Delay  en=off  latency=1  dbl_ovrd=off  reg_retiming=off  block_type=delay
      settings: xl_area=[1 1 0 0 0 0 0]  block_version=12.1
  Out1 : Outport
  Out2 : Outport  Port=2
  wires:
  1to2/2(Out2) -> Out2/1
  1to2/1(Out1) -> Out1/1
  In1/1 -> DE/1
  DE/1 -> 1to2/1(In)

== system receiver_overall_reset/Receiver/Sym-Chooser/2-10/Corr0/Delay_Line/DE29 ==
  In1 : Inport
  1to2 : Subsystem
  DE : xbsIndex_r4/Delay  en=off  latency=1  dbl_ovrd=off  reg_retiming=off  block_type=delay
      settings: xl_area=[1 1 0 0 0 0 0]  block_version=12.1
  Out1 : Outport
  Out2 : Outport  Port=2
  wires:
  1to2/2(Out2) -> Out2/1
  1to2/1(Out1) -> Out1/1
  In1/1 -> DE/1
  DE/1 -> 1to2/1(In)

== system receiver_overall_reset/Receiver/Sym-Chooser/2-10/Corr0/Delay_Line/DE3 ==
  In1 : Inport
  1to2 : Subsystem
  DE : xbsIndex_r4/Delay  en=off  latency=1  dbl_ovrd=off  reg_retiming=off  block_type=delay
      settings: xl_area=[1 1 0 0 0 0 0]  block_version=12.1
  Out1 : Outport
  Out2 : Outport  Port=2
  wires:
  1to2/2(Out2) -> Out2/1
  1to2/1(Out1) -> Out1/1
  In1/1 -> DE/1
  DE/1 -> 1to2/1(In)

== system receiver_overall_reset/Receiver/Sym-Chooser/2-10/Corr0/Delay_Line/DE30 ==
  In1 : Inport
  1to2 : Subsystem
  DE : xbsIndex_r4/Delay  en=off  latency=1  dbl_ovrd=off  reg_retiming=off  block_type=delay
      settings: xl_area=[1 1 0 0 0 0 0]  block_version=12.1
  Out1 : Outport
  Out2 : Outport  Port=2
  wires:
  1to2/2(Out2) -> Out2/1
  1to2/1(Out1) -> Out1/1
  In1/1 -> DE/1
  DE/1 -> 1to2/1(In)

== system receiver_overall_reset/Receiver/Sym-Chooser/2-10/Corr0/Delay_Line/DE4 ==
  In1 : Inport
  1to2 : Subsystem
  DE : xbsIndex_r4/Delay  en=off  latency=1  dbl_ovrd=off  reg_retiming=off  block_type=delay
      settings: xl_area=[1 1 0 0 0 0 0]  block_version=12.1
  Out1 : Outport
  Out2 : Outport  Port=2
  wires:
  1to2/2(Out2) -> Out2/1
  1to2/1(Out1) -> Out1/1
  In1/1 -> DE/1
  DE/1 -> 1to2/1(In)

== system receiver_overall_reset/Receiver/Sym-Chooser/2-10/Corr0/Delay_Line/DE5 ==
  In1 : Inport
  1to2 : Subsystem
  DE : xbsIndex_r4/Delay  en=off  latency=1  dbl_ovrd=off  reg_retiming=off  block_type=delay
      settings: xl_area=[1 1 0 0 0 0 0]  block_version=12.1
  Out1 : Outport
  Out2 : Outport  Port=2
  wires:
  1to2/2(Out2) -> Out2/1
  1to2/1(Out1) -> Out1/1
  In1/1 -> DE/1
  DE/1 -> 1to2/1(In)

== system receiver_overall_reset/Receiver/Sym-Chooser/2-10/Corr0/Delay_Line/DE6 ==
  In1 : Inport
  1to2 : Subsystem
  DE : xbsIndex_r4/Delay  en=off  latency=1  dbl_ovrd=off  reg_retiming=off  block_type=delay
      settings: xl_area=[1 1 0 0 0 0 0]  block_version=12.1
  Out1 : Outport
  Out2 : Outport  Port=2
  wires:
  1to2/2(Out2) -> Out2/1
  1to2/1(Out1) -> Out1/1
  In1/1 -> DE/1
  DE/1 -> 1to2/1(In)

== system receiver_overall_reset/Receiver/Sym-Chooser/2-10/Corr0/Delay_Line/DE7 ==
  In1 : Inport
  1to2 : Subsystem
  DE : xbsIndex_r4/Delay  en=off  latency=1  dbl_ovrd=off  reg_retiming=off  block_type=delay
      settings: xl_area=[1 1 0 0 0 0 0]  block_version=12.1
  Out1 : Outport
  Out2 : Outport  Port=2
  wires:
  1to2/2(Out2) -> Out2/1
  1to2/1(Out1) -> Out1/1
  In1/1 -> DE/1
  DE/1 -> 1to2/1(In)

== system receiver_overall_reset/Receiver/Sym-Chooser/2-10/Corr0/Delay_Line/DE8 ==
  In1 : Inport
  1to2 : Subsystem
  DE : xbsIndex_r4/Delay  en=off  latency=1  dbl_ovrd=off  reg_retiming=off  block_type=delay
      settings: xl_area=[1 1 0 0 0 0 0]  block_version=12.1
  Out1 : Outport
  Out2 : Outport  Port=2
  wires:
  1to2/2(Out2) -> Out2/1
  1to2/1(Out1) -> Out1/1
  In1/1 -> DE/1
  DE/1 -> 1to2/1(In)

== system receiver_overall_reset/Receiver/Sym-Chooser/2-10/Corr0/Delay_Line/DE9 ==
  In1 : Inport
  1to2 : Subsystem
  DE : xbsIndex_r4/Delay  en=off  latency=1  dbl_ovrd=off  reg_retiming=off  block_type=delay
      settings: xl_area=[1 1 0 0 0 0 0]  block_version=12.1
  Out1 : Outport
  Out2 : Outport  Port=2
  wires:
  1to2/2(Out2) -> Out2/1
  1to2/1(Out1) -> Out1/1
  In1/1 -> DE/1
  DE/1 -> 1to2/1(In)

== system receiver_overall_reset/Receiver/Sym-Chooser/3-11/Corr0/Delay_Line/1to2 ==
  In : Inport  OutDataType=fixdt(1, 16)  OutScaling=2^0
  Out1 : Outport  OutDataType=fixdt(1, 16)  OutScaling=2^0
  Out2 : Outport  Port=2  OutDataType=fixdt(1, 16)  OutScaling=2^0
  wires:
  In/1 -> Out1/1, Out2/1

== system receiver_overall_reset/Receiver/Sym-Chooser/3-11/Corr0/Delay_Line/DE1 ==
  In1 : Inport
  1to2 : Subsystem
  DE : xbsIndex_r4/Delay  en=off  latency=1  dbl_ovrd=off  reg_retiming=off  block_type=delay
      settings: xl_area=[1 1 0 0 0 0 0]  block_version=12.1
  Out1 : Outport
  Out2 : Outport  Port=2
  wires:
  DE/1 -> 1to2/1(In)
  In1/1 -> DE/1
  1to2/1(Out1) -> Out1/1
  1to2/2(Out2) -> Out2/1

== system receiver_overall_reset/Receiver/Sym-Chooser/3-11/Corr0/Delay_Line/DE10 ==
  In1 : Inport
  1to2 : Subsystem
  DE : xbsIndex_r4/Delay  en=off  latency=1  dbl_ovrd=off  reg_retiming=off  block_type=delay
      settings: xl_area=[1 1 0 0 0 0 0]  block_version=12.1
  Out1 : Outport
  Out2 : Outport  Port=2
  wires:
  1to2/2(Out2) -> Out2/1
  1to2/1(Out1) -> Out1/1
  In1/1 -> DE/1
  DE/1 -> 1to2/1(In)

== system receiver_overall_reset/Receiver/Sym-Chooser/3-11/Corr0/Delay_Line/DE11 ==
  In1 : Inport
  1to2 : Subsystem
  DE : xbsIndex_r4/Delay  en=off  latency=1  dbl_ovrd=off  reg_retiming=off  block_type=delay
      settings: xl_area=[1 1 0 0 0 0 0]  block_version=12.1
  Out1 : Outport
  Out2 : Outport  Port=2
  wires:
  1to2/2(Out2) -> Out2/1
  1to2/1(Out1) -> Out1/1
  In1/1 -> DE/1
  DE/1 -> 1to2/1(In)

== system receiver_overall_reset/Receiver/Sym-Chooser/3-11/Corr0/Delay_Line/DE12 ==
  In1 : Inport
  1to2 : Subsystem
  DE : xbsIndex_r4/Delay  en=off  latency=1  dbl_ovrd=off  reg_retiming=off  block_type=delay
      settings: xl_area=[1 1 0 0 0 0 0]  block_version=12.1
  Out1 : Outport
  Out2 : Outport  Port=2
  wires:
  1to2/2(Out2) -> Out2/1
  1to2/1(Out1) -> Out1/1
  In1/1 -> DE/1
  DE/1 -> 1to2/1(In)

== system receiver_overall_reset/Receiver/Sym-Chooser/3-11/Corr0/Delay_Line/DE13 ==
  In1 : Inport
  1to2 : Subsystem
  DE : xbsIndex_r4/Delay  en=off  latency=1  dbl_ovrd=off  reg_retiming=off  block_type=delay
      settings: xl_area=[1 1 0 0 0 0 0]  block_version=12.1
  Out1 : Outport
  Out2 : Outport  Port=2
  wires:
  1to2/2(Out2) -> Out2/1
  1to2/1(Out1) -> Out1/1
  In1/1 -> DE/1
  DE/1 -> 1to2/1(In)
